simulink model "Even_Odd"  (R2021a)
settings: Solver=FixedStepDiscrete  StartTime=0.0  StopTime=10.0  RelTol=1e-3
settings Model: Creator=Moamen_Hamed  LastModifiedBy=Moamen_Hamed
settings OptimizationCC: DefaultParameterBehavior=Inlined  EnhancedBackFolding=on  PassReuseOutputArgsAs=Individual arguments  OptimizeBlockOrder=speed  DifferentSizesBufferReuse=on  OptimizationCustomize=off  EfficientTunableParamExpr=on
settings DebuggingCC: ParameterTunabilityLossMsg=error
settings SFSimCC: MATLABDynamicMemAlloc=off
settings RTWCC: SystemTargetFile=ert.tlc  GenCodeOnly=on  TemplateMakefile=ert_default_tmf  GenerateReport=on  IncludeHyperlinkInReport=on  LaunchReport=on  GenerateTraceInfo=on
settings CodeAppCC: ForceParamTrailComments=on  IgnoreCustomStorageClasses=off  OperatorAnnotations=on  SimulinkDataObjDesc=on  SFDataObjDesc=on  InsertBlockDesc=on
settings ERTTargetCC: TargetLangStandard=C99 (ISO)  GenerateSampleERTMain=on  CodeInterfacePackaging=Reusable function  SupportComplex=off  InlinedParameterPlacement=NonHierarchical  ERTCustomFileTemplate=example_file_process.tlc

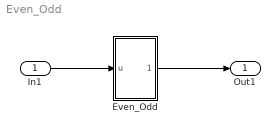
== system Even_Odd ==
  In1 : Inport
  Even_Odd : Subsystem  TreatAsAtomicUnit=on
  Out1 : Outport
  wires:
  In1/1 -> Even_Odd/1(u)
  Even_Odd/1(Out1) -> Out1/1

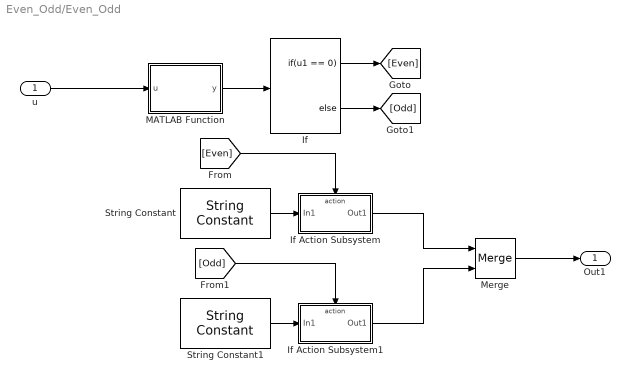
== system Even_Odd/Even_Odd ==
  u : Inport
  If : If  IfExpression=u1 == 0
  If Action Subsystem : Subsystem  TreatAsAtomicUnit=on
  If Action Subsystem1 : Subsystem  TreatAsAtomicUnit=on
  MATLAB Function : MATLAB Function  TreatAsAtomicUnit=on
  Merge : Merge
  String Constant : StringConstant  String="\"The number is even!\""
  String Constant1 : StringConstant  String="\"The number is odd!\""
  Out1 : Outport
  wires:
  If/1 -> [Even]
  String Constant/1 -> If Action Subsystem/1(In1)
  If Action Subsystem/1(Out1) -> Merge/1
  [Odd] -> If Action Subsystem1/Action
  [Even] -> If Action Subsystem/Action
  MATLAB Function/1(y) -> If/1
  If Action Subsystem1/1(Out1) -> Merge/2
  If/2 -> [Odd]
  String Constant1/1 -> If Action Subsystem1/1(In1)
  Merge/1 -> Out1/1
  u/1 -> MATLAB Function/1(u)

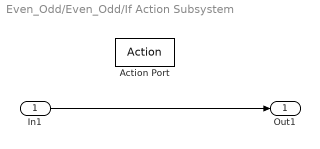
== system Even_Odd/Even_Odd/If Action Subsystem ==
  In1 : Inport
  Action Port : ActionPort  ActionPortLabel=if(u1 == 0)
  Out1 : Outport
  wires:
  In1/1 -> Out1/1

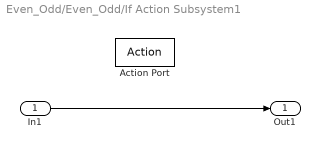
== system Even_Odd/Even_Odd/If Action Subsystem1 ==
  In1 : Inport
  Action Port : ActionPort  ActionPortLabel=else
  Out1 : Outport
  wires:
  In1/1 -> Out1/1

== matlab function Even_Odd/MATLAB Function ==
  data: u input; y output
function y = Even_odd(u)
if rem(u,2) == 0 
y = 0;  
else 
y = 1;  
end
